simulink model "Final_Input_dat_rev1"  (R2024a)
settings: Solver=VariableStepAuto  StartTime=0.0  StopTime=10.0  RelTol=1e-3
libraries: CarMaker4SL x58
settings Model: Creator=namwoo.kim  LastModifiedBy=namwoo.kim

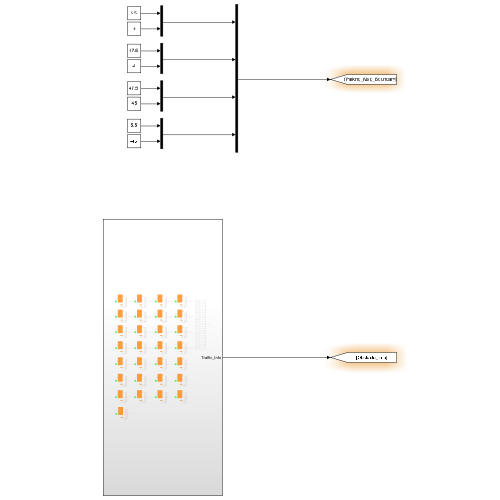
[thumbnail: Simulink's stored preview of the top-level diagram]
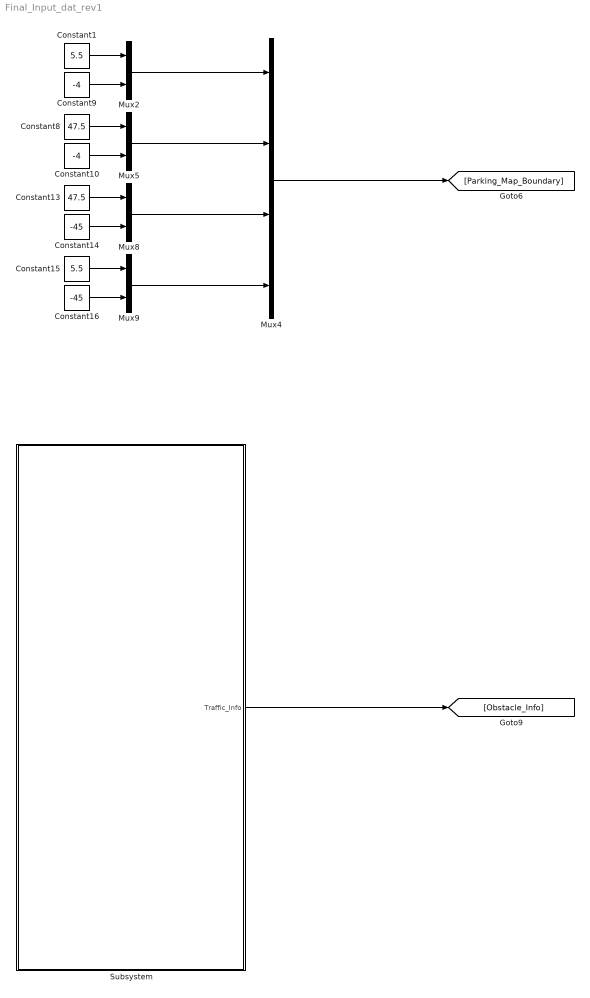
== system Final_Input_dat_rev1 ==
  Constant1 : Constant  Value=5.5
  Constant10 : Constant  Value=-4
  Constant13 : Constant  Value=47.5
  Constant14 : Constant  Value=-45
  Constant15 : Constant  Value=5.5
  Constant16 : Constant  Value=-45
  Constant8 : Constant  Value=47.5
  Constant9 : Constant  Value=-4
  Mux{2,5,8..9} (4 alike) : Mux  Inputs=2
  Mux4 : Mux
  Subsystem : Subsystem
  wires:
  Constant8/1 -> Mux5/1
  Constant16/1 -> Mux9/2
  Constant10/1 -> Mux5/2
  Mux4/1 -> [Parking_Map_Boundary]
  Constant15/1 -> Mux9/1
  Constant1/1 -> Mux2/1
  Mux8/1 -> Mux4/3
  Mux2/1 -> Mux4/1
  Mux5/1 -> Mux4/2
  Constant13/1 -> Mux8/1
  Constant9/1 -> Mux2/2
  Subsystem/1(Traffic_Info) -> [Obstacle_Info]
  Mux9/1 -> Mux4/4
  Constant14/1 -> Mux8/2

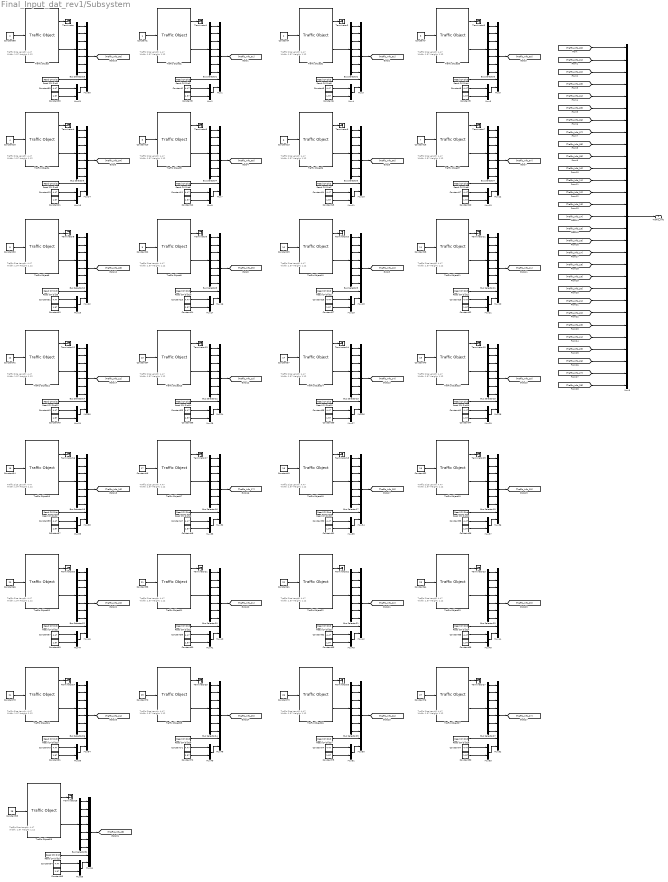
== system Final_Input_dat_rev1/Subsystem ==
  note: Traffic Size
      | Length: 4.47
      | Width: 1.97
      | Height: 1.12
  note: Traffic Size
      | Length: 4.47
      | Width: 1.97
      | Height: 1.12
  note: Traffic Size
      | Length: 4.47
      | Width: 1.97
      | Height: 1.12
  note: Traffic Size
      | Length: 4.47
      | Width: 1.97
      | Height: 1.12
  note: Traffic Size
      | Length: 4.47
      | Width: 1.97
      | Height: 1.12
  note: Traffic Size
      | Length: 4.47
      | Width: 1.97
      | Height: 1.12
  note: Traffic Size
      | Length: 4.47
      | Width: 1.97
      | Height: 1.12
  note: Traffic Size
      | Length: 4.47
      | Width: 1.97
      | Height: 1.12
  note: Traffic Size
      | Length: 4.47
      | Width: 1.97
      | Height: 1.12
  note: Traffic Size
      | Length: 4.47
      | Width: 1.97
      | Height: 1.12
  note: Traffic Size
      | Length: 4.47
      | Width: 1.97
      | Height: 1.12
  note: Traffic Size
      | Length: 4.47
      | Width: 1.97
      | Height: 1.12
  note: Traffic Size
      | Length: 4.47
      | Width: 1.97
      | Height: 1.12
  note: Traffic Size
      | Length: 4.47
      | Width: 1.97
      | Height: 1.12
  note: Traffic Size
      | Length: 4.47
      | Width: 1.97
      | Height: 1.12
  note: Traffic Size
      | Length: 4.47
      | Width: 1.97
      | Height: 1.12
  note: Traffic Size
      | Length: 4.47
      | Width: 1.97
      | Height: 1.12
  note: Traffic Size
      | Length: 4.47
      | Width: 1.97
      | Height: 1.12
  note: Traffic Size
      | Length: 4.47
      | Width: 1.97
      | Height: 1.12
  note: Traffic Size
      | Length: 4.47
      | Width: 1.97
      | Height: 1.12
  note: Traffic Size
      | Length: 4.47
      | Width: 1.97
      | Height: 1.12
  note: Traffic Size
      | Length: 4.47
      | Width: 1.97
      | Height: 1.12
  note: Traffic Size
      | Length: 4.47
      | Width: 1.97
      | Height: 1.12
  note: Traffic Size
      | Length: 4.47
      | Width: 1.97
      | Height: 1.12
  note: Traffic Size
      | Length: 4.47
      | Width: 1.97
      | Height: 1.12
  note: Traffic Size
      | Length: 4.47
      | Width: 1.97
      | Height: 1.12
  note: Traffic Size
      | Length: 4.47
      | Width: 1.97
      | Height: 1.12
  note: Traffic Size
      | Length: 4.47
      | Width: 1.97
      | Height: 1.12
  note: Traffic Size
      | Length: 4.47
      | Width: 1.97
      | Height: 1.12
  Bus Selector{1..27,29,31} (29 alike) : BusSelector  OutputSignals=t_0 x,t_0 y,v_0 x,v_0 y,a_0 x,a_0 y,r_zyx z
  Constant1 : Constant
  Constant10 : Constant  Value=5
  Constant{2,5,8,11,14,17,19,23,26,29,31,35,38,41,43,47,50,53,55,59,62,65,67,71,74,77,79,89,94} (29 alike) : Constant  Value=4.47
  Constant{3,6,9,12,15,20..21,24,27,32..33,36,39,44..45,48,51,56..57,60,63,68..69,72,75,80..81,90,96} (29 alike) : Constant  Value=1.97
  Constant13 : Constant  Value=6
  Constant16 : Constant  Value=7
  Constant18 : Constant  Value=4
  Constant22 : Constant  Value=9
  Constant25 : Constant  Value=10
  Constant28 : Constant  Value=11
  Constant30 : Constant  Value=8
  Constant34 : Constant  Value=13
  Constant37 : Constant  Value=14
  Constant4 : Constant  Value=2
  Constant40 : Constant  Value=15
  Constant42 : Constant  Value=12
  Constant46 : Constant  Value=17
  Constant49 : Constant  Value=18
  Constant52 : Constant  Value=19
  Constant54 : Constant  Value=16
  Constant58 : Constant  Value=21
  Constant61 : Constant  Value=22
  Constant64 : Constant  Value=23
  Constant66 : Constant  Value=20
  Constant7 : Constant  Value=3
  Constant70 : Constant  Value=25
  Constant73 : Constant  Value=26
  Constant76 : Constant  Value=27
  Constant78 : Constant  Value=24
  Constant88 : Constant  Value=0
  Constant93 : Constant  Value=28
  Mux{1,3,5,7,10,12,14,16,18,20,22,24,26,28,30,32,34,36,38,40,42,44,46,48,50,52,54,60,64} (29 alike) : Mux  Inputs=9
  Mux{2,4,6,8,11,13,15,17,19,21,23,25,27,29,31,33,35,37,39,41,43,45,47,49,51,53,55,61,65} (29 alike) : Mux  Inputs=2
  Mux9 : Mux  Inputs=29
  Read CM Dict1 : CarMaker4SL/Read CM Dict  xname=Traffic.T00.rzv  xsync=off  xstime=Inherited
  Read CM Dict10 : CarMaker4SL/Read CM Dict  xname=Traffic.T09.rzv  xsync=off  xstime=Inherited
  Read CM Dict11 : CarMaker4SL/Read CM Dict  xname=Traffic.T10.rzv  xsync=off  xstime=Inherited
  Read CM Dict12 : CarMaker4SL/Read CM Dict  xname=Traffic.T11.rzv  xsync=off  xstime=Inherited
  Read CM Dict13 : CarMaker4SL/Read CM Dict  xname=Traffic.T12.rzv  xsync=off  xstime=Inherited
  Read CM Dict14 : CarMaker4SL/Read CM Dict  xname=Traffic.T13.rzv  xsync=off  xstime=Inherited
  Read CM Dict15 : CarMaker4SL/Read CM Dict  xname=Traffic.T14.rzv  xsync=off  xstime=Inherited
  Read CM Dict16 : CarMaker4SL/Read CM Dict  xname=Traffic.T15.rzv  xsync=off  xstime=Inherited
  Read CM Dict17 : CarMaker4SL/Read CM Dict  xname=Traffic.T16.rzv  xsync=off  xstime=Inherited
  Read CM Dict18 : CarMaker4SL/Read CM Dict  xname=Traffic.T17.rzv  xsync=off  xstime=Inherited
  Read CM Dict19 : CarMaker4SL/Read CM Dict  xname=Traffic.T18.rzv  xsync=off  xstime=Inherited
  Read CM Dict2 : CarMaker4SL/Read CM Dict  xname=Traffic.T01.rzv  xsync=off  xstime=Inherited
  Read CM Dict20 : CarMaker4SL/Read CM Dict  xname=Traffic.T15.rzv  xsync=off  xstime=Inherited
  Read CM Dict21 : CarMaker4SL/Read CM Dict  xname=Traffic.T20.rzv  xsync=off  xstime=Inherited
  Read CM Dict22 : CarMaker4SL/Read CM Dict  xname=Traffic.T21.rzv  xsync=off  xstime=Inherited
  Read CM Dict23 : CarMaker4SL/Read CM Dict  xname=Traffic.T22.rzv  xsync=off  xstime=Inherited
  Read CM Dict24 : CarMaker4SL/Read CM Dict  xname=Traffic.T23.rzv  xsync=off  xstime=Inherited
  Read CM Dict25 : CarMaker4SL/Read CM Dict  xname=Traffic.T24.rzv  xsync=off  xstime=Inherited
  Read CM Dict26 : CarMaker4SL/Read CM Dict  xname=Traffic.T25.rzv  xsync=off  xstime=Inherited
  Read CM Dict27 : CarMaker4SL/Read CM Dict  xname=Traffic.T26.rzv  xsync=off  xstime=Inherited
  Read CM Dict28 : CarMaker4SL/Read CM Dict  xname=Traffic.T27.rzv  xsync=off  xstime=Inherited
  Read CM Dict29 : CarMaker4SL/Read CM Dict  xname=Traffic.T28.rzv  xsync=off  xstime=Inherited
  Read CM Dict3 : CarMaker4SL/Read CM Dict  xname=Traffic.T02.rzv  xsync=off  xstime=Inherited
  Read CM Dict4 : CarMaker4SL/Read CM Dict  xname=Traffic.T03.rzv  xsync=off  xstime=Inherited
  Read CM Dict5 : CarMaker4SL/Read CM Dict  xname=Traffic.T04.rzv  xsync=off  xstime=Inherited
  Read CM Dict6 : CarMaker4SL/Read CM Dict  xname=Traffic.T05.rzv  xsync=off  xstime=Inherited
  Read CM Dict7 : CarMaker4SL/Read CM Dict  xname=Traffic.T06.rzv  xsync=off  xstime=Inherited
  Read CM Dict8 : CarMaker4SL/Read CM Dict  xname=Traffic.T07.rzv  xsync=off  xstime=Inherited
  Read CM Dict9 : CarMaker4SL/Read CM Dict  xname=Traffic.T08.rzv  xsync=off  xstime=Inherited
  Terminator{,1..28} (29 alike) : Terminator
  Traffic Object : CarMaker4SL/Traffic Object  xname=T00  ximode=Traffic Id  xstime=Inherited
      settings: SourceProductName=CarMaker4SL
  Traffic Object1 : CarMaker4SL/Traffic Object  xname=T01  ximode=Traffic Id  xstime=Inherited
      settings: SourceProductName=CarMaker4SL
  Traffic Object10 : CarMaker4SL/Traffic Object  xname=T10  ximode=Traffic Id  xstime=Inherited
      settings: SourceProductName=CarMaker4SL
  Traffic Object11 : CarMaker4SL/Traffic Object  xname=T11  ximode=Traffic Id  xstime=Inherited
      settings: SourceProductName=CarMaker4SL
  Traffic Object12 : CarMaker4SL/Traffic Object  xname=T12  ximode=Traffic Id  xstime=Inherited
      settings: SourceProductName=CarMaker4SL
  Traffic Object13 : CarMaker4SL/Traffic Object  xname=T13  ximode=Traffic Id  xstime=Inherited
      settings: SourceProductName=CarMaker4SL
  Traffic Object14 : CarMaker4SL/Traffic Object  xname=T14  ximode=Traffic Id  xstime=Inherited
      settings: SourceProductName=CarMaker4SL
  Traffic Object15 : CarMaker4SL/Traffic Object  xname=T15  ximode=Traffic Id  xstime=Inherited
      settings: SourceProductName=CarMaker4SL
  Traffic Object16 : CarMaker4SL/Traffic Object  xname=T16  ximode=Traffic Id  xstime=Inherited
      settings: SourceProductName=CarMaker4SL
  Traffic Object17 : CarMaker4SL/Traffic Object  xname=T17  ximode=Traffic Id  xstime=Inherited
      settings: SourceProductName=CarMaker4SL
  Traffic Object18 : CarMaker4SL/Traffic Object  xname=T18  ximode=Traffic Id  xstime=Inherited
      settings: SourceProductName=CarMaker4SL
  Traffic Object19 : CarMaker4SL/Traffic Object  xname=T19  ximode=Traffic Id  xstime=Inherited
      settings: SourceProductName=CarMaker4SL
  Traffic Object2 : CarMaker4SL/Traffic Object  xname=T02  ximode=Traffic Id  xstime=Inherited
      settings: SourceProductName=CarMaker4SL
  Traffic Object20 : CarMaker4SL/Traffic Object  xname=T20  ximode=Traffic Id  xstime=Inherited
      settings: SourceProductName=CarMaker4SL
  Traffic Object21 : CarMaker4SL/Traffic Object  xname=T21  ximode=Traffic Id  xstime=Inherited
      settings: SourceProductName=CarMaker4SL
  Traffic Object22 : CarMaker4SL/Traffic Object  xname=T22  ximode=Traffic Id  xstime=Inherited
      settings: SourceProductName=CarMaker4SL
  Traffic Object23 : CarMaker4SL/Traffic Object  xname=T23  ximode=Traffic Id  xstime=Inherited
      settings: SourceProductName=CarMaker4SL
  Traffic Object24 : CarMaker4SL/Traffic Object  xname=T24  ximode=Traffic Id  xstime=Inherited
      settings: SourceProductName=CarMaker4SL
  Traffic Object25 : CarMaker4SL/Traffic Object  xname=T25  ximode=Traffic Id  xstime=Inherited
      settings: SourceProductName=CarMaker4SL
  Traffic Object26 : CarMaker4SL/Traffic Object  xname=T26  ximode=Traffic Id  xstime=Inherited
      settings: SourceProductName=CarMaker4SL
  Traffic Object27 : CarMaker4SL/Traffic Object  xname=T27  ximode=Traffic Id  xstime=Inherited
      settings: SourceProductName=CarMaker4SL
  Traffic Object28 : CarMaker4SL/Traffic Object  xname=T28  ximode=Traffic Id  xstime=Inherited
      settings: SourceProductName=CarMaker4SL
  Traffic Object3 : CarMaker4SL/Traffic Object  xname=T03  ximode=Traffic Id  xstime=Inherited
      settings: SourceProductName=CarMaker4SL
  Traffic Object4 : CarMaker4SL/Traffic Object  xname=T04  ximode=Traffic Id  xstime=Inherited
      settings: SourceProductName=CarMaker4SL
  Traffic Object5 : CarMaker4SL/Traffic Object  xname=T05  ximode=Traffic Id  xstime=Inherited
      settings: SourceProductName=CarMaker4SL
  Traffic Object6 : CarMaker4SL/Traffic Object  xname=T06  ximode=Traffic Id  xstime=Inherited
      settings: SourceProductName=CarMaker4SL
  Traffic Object7 : CarMaker4SL/Traffic Object  xname=T07  ximode=Traffic Id  xstime=Inherited
      settings: SourceProductName=CarMaker4SL
  Traffic Object8 : CarMaker4SL/Traffic Object  xname=T08  ximode=Traffic Id  xstime=Inherited
      settings: SourceProductName=CarMaker4SL
  Traffic Object9 : CarMaker4SL/Traffic Object  xname=T09  ximode=Traffic Id  xstime=Inherited
      settings: SourceProductName=CarMaker4SL
  Traffic_Info : Outport
  wires:
  [Traffic_Info_00] -> Mux9/1
  [Traffic_Info_01] -> Mux9/2
  Mux9/1 -> Traffic_Info/1
  [Traffic_Info_02] -> Mux9/3
  [Traffic_Info_06] -> Mux9/7
  [Traffic_Info_05] -> Mux9/6
  [Traffic_Info_04] -> Mux9/5
  [Traffic_Info_03] -> Mux9/4
  [Traffic_Info_09] -> Mux9/10
  [Traffic_Info_10] -> Mux9/11
  [Traffic_Info_11] -> Mux9/12
  [Traffic_Info_08] -> Mux9/9
  [Traffic_Info_12] -> Mux9/13
  [Traffic_Info_13] -> Mux9/14
  [Traffic_Info_07] -> Mux9/8
  [Traffic_Info_16] -> Mux9/17
  [Traffic_Info_17] -> Mux9/18
  [Traffic_Info_18] -> Mux9/19
  [Traffic_Info_15] -> Mux9/16
  [Traffic_Info_19] -> Mux9/20
  [Traffic_Info_20] -> Mux9/21
  [Traffic_Info_14] -> Mux9/15
  [Traffic_Info_23] -> Mux9/24
  [Traffic_Info_24] -> Mux9/25
  [Traffic_Info_25] -> Mux9/26
  [Traffic_Info_22] -> Mux9/23
  [Traffic_Info_26] -> Mux9/27
  [Traffic_Info_27] -> Mux9/28
  [Traffic_Info_21] -> Mux9/22
  [Traffic_Info_28] -> Mux9/29
  Traffic Object/2 -> Bus Selector29/1
  Constant88/1 -> Traffic Object/1
  Traffic Object/1 -> Terminator/1
  Bus Selector29/1 -> Mux60/1  "<t_0 x>"
  Bus Selector29/2 -> Mux60/2  "<t_0 y>"
  Bus Selector29/4 -> Mux60/4  "<v_0 y>"
  Bus Selector29/5 -> Mux60/5  "<a_0 x>"
  Bus Selector29/3 -> Mux60/3  "<v_0 x>"
  Bus Selector29/6 -> Mux60/6  "<a_0 y>"
  Bus Selector29/7 -> Mux60/7  "<r_zyx z>"
  Read CM Dict1/1 -> Mux60/8
  Mux60/1 -> [Traffic_Info_00]
  Constant89/1 -> Mux61/1
  Constant90/1 -> Mux61/2
  Mux61/1 -> Mux60/9
  Mux2/1 -> Mux1/9
  Constant2/1 -> Mux2/1
  Constant3/1 -> Mux2/2
  Bus Selector1/2 -> Mux1/2  "<t_0 y>"
  Traffic Object1/2 -> Bus Selector1/1
  Traffic Object1/1 -> Terminator1/1
  Constant1/1 -> Traffic Object1/1
  Read CM Dict2/1 -> Mux1/8
  Bus Selector1/1 -> Mux1/1  "<t_0 x>"
  Bus Selector1/6 -> Mux1/6  "<a_0 y>"
  Bus Selector1/7 -> Mux1/7  "<r_zyx z>"
  Bus Selector1/4 -> Mux1/4  "<v_0 y>"
  Bus Selector1/5 -> Mux1/5  "<a_0 x>"
  Mux1/1 -> [Traffic_Info_01]
  Bus Selector1/3 -> Mux1/3  "<v_0 x>"
  Mux4/1 -> Mux3/9
  Constant5/1 -> Mux4/1
  Constant6/1 -> Mux4/2
  Bus Selector2/2 -> Mux3/2  "<t_0 y>"
  Traffic Object2/2 -> Bus Selector2/1
  Traffic Object2/1 -> Terminator2/1
  Constant4/1 -> Traffic Object2/1
  Read CM Dict3/1 -> Mux3/8
  Bus Selector2/1 -> Mux3/1  "<t_0 x>"
  Bus Selector2/6 -> Mux3/6  "<a_0 y>"
  Bus Selector2/7 -> Mux3/7  "<r_zyx z>"
  Bus Selector2/4 -> Mux3/4  "<v_0 y>"
  Bus Selector2/5 -> Mux3/5  "<a_0 x>"
  Mux3/1 -> [Traffic_Info_02]
  Bus Selector2/3 -> Mux3/3  "<v_0 x>"
  Mux6/1 -> Mux5/9
  Constant8/1 -> Mux6/1
  Constant9/1 -> Mux6/2
  Bus Selector3/2 -> Mux5/2  "<t_0 y>"
  Traffic Object3/2 -> Bus Selector3/1
  Traffic Object3/1 -> Terminator3/1
  Constant7/1 -> Traffic Object3/1
  Read CM Dict4/1 -> Mux5/8
  Bus Selector3/1 -> Mux5/1  "<t_0 x>"
  Bus Selector3/6 -> Mux5/6  "<a_0 y>"
  Bus Selector3/7 -> Mux5/7  "<r_zyx z>"
  Bus Selector3/4 -> Mux5/4  "<v_0 y>"
  Bus Selector3/5 -> Mux5/5  "<a_0 x>"
  Mux5/1 -> [Traffic_Info_03]
  Bus Selector3/3 -> Mux5/3  "<v_0 x>"
  Constant19/1 -> Mux15/1
  Constant21/1 -> Mux15/2
  Bus Selector4/3 -> Mux7/3  "<v_0 x>"
  Bus Selector4/4 -> Mux7/4  "<v_0 y>"
  Bus Selector4/7 -> Mux7/7  "<r_zyx z>"
  Read CM Dict6/1 -> Mux7/8
  Traffic Object5/1 -> Terminator5/1
  Mux15/1 -> Mux14/9
  Bus Selector4/2 -> Mux7/2  "<t_0 y>"
  Constant11/1 -> Mux8/1
  Constant12/1 -> Mux8/2
  Bus Selector4/1 -> Mux7/1  "<t_0 x>"
  Bus Selector5/3 -> Mux10/3  "<v_0 x>"
  Bus Selector5/4 -> Mux10/4  "<v_0 y>"
  Bus Selector5/7 -> Mux10/7  "<r_zyx z>"
  Traffic Object4/1 -> Terminator4/1
  Constant18/1 -> Traffic Object4/1
  Bus Selector5/1 -> Mux10/1  "<t_0 x>"
  Bus Selector5/6 -> Mux10/6  "<a_0 y>"
  Traffic Object4/2 -> Bus Selector6/1
  Bus Selector7/3 -> Mux12/3  "<v_0 x>"
  Bus Selector6/2 -> Mux14/2  "<t_0 y>"
  Mux7/1 -> [Traffic_Info_05]
  Bus Selector7/4 -> Mux12/4  "<v_0 y>"
  Mux12/1 -> [Traffic_Info_07]
  Traffic Object7/2 -> Bus Selector7/1
  Read CM Dict8/1 -> Mux12/8
  Constant16/1 -> Traffic Object7/1
  Read CM Dict5/1 -> Mux14/8
  Mux13/1 -> Mux12/9
  Bus Selector4/6 -> Mux7/6  "<a_0 y>"
  Constant20/1 -> Mux13/2
  Constant10/1 -> Traffic Object5/1
  Bus Selector7/7 -> Mux12/7  "<r_zyx z>"
  Traffic Object5/2 -> Bus Selector4/1
  Traffic Object7/1 -> Terminator7/1
  Bus Selector6/1 -> Mux14/1  "<t_0 x>"
  Bus Selector6/7 -> Mux14/7  "<r_zyx z>"
  Bus Selector7/6 -> Mux12/6  "<a_0 y>"
  Bus Selector6/4 -> Mux14/4  "<v_0 y>"
  Constant13/1 -> Traffic Object6/1
  Bus Selector5/5 -> Mux10/5  "<a_0 x>"
  Traffic Object6/1 -> Terminator6/1
  Read CM Dict7/1 -> Mux10/8
  Bus Selector5/2 -> Mux10/2  "<t_0 y>"
  Bus Selector7/1 -> Mux12/1  "<t_0 x>"
  Constant14/1 -> Mux11/1
  Bus Selector7/2 -> Mux12/2  "<t_0 y>"
  Mux8/1 -> Mux7/9
  Constant15/1 -> Mux11/2
  Bus Selector4/5 -> Mux7/5  "<a_0 x>"
  Traffic Object6/2 -> Bus Selector5/1
  Bus Selector6/6 -> Mux14/6  "<a_0 y>"
  Bus Selector6/5 -> Mux14/5  "<a_0 x>"
  Bus Selector7/5 -> Mux12/5  "<a_0 x>"
  Mux11/1 -> Mux10/9
  Mux14/1 -> [Traffic_Info_04]
  Constant17/1 -> Mux13/1
  Bus Selector6/3 -> Mux14/3  "<v_0 x>"
  Mux10/1 -> [Traffic_Info_06]
  Constant31/1 -> Mux23/1
  Constant33/1 -> Mux23/2
  Bus Selector8/3 -> Mux16/3  "<v_0 x>"
  Bus Selector8/4 -> Mux16/4  "<v_0 y>"
  Bus Selector8/7 -> Mux16/7  "<r_zyx z>"
  Read CM Dict10/1 -> Mux16/8
  Traffic Object9/1 -> Terminator9/1
  Mux23/1 -> Mux22/9
  Bus Selector8/2 -> Mux16/2  "<t_0 y>"
  Constant23/1 -> Mux17/1
  Constant24/1 -> Mux17/2
  Bus Selector8/1 -> Mux16/1  "<t_0 x>"
  Bus Selector9/3 -> Mux18/3  "<v_0 x>"
  Bus Selector9/4 -> Mux18/4  "<v_0 y>"
  Bus Selector9/7 -> Mux18/7  "<r_zyx z>"
  Traffic Object8/1 -> Terminator8/1
  Constant30/1 -> Traffic Object8/1
  Bus Selector9/1 -> Mux18/1  "<t_0 x>"
  Bus Selector9/6 -> Mux18/6  "<a_0 y>"
  Traffic Object8/2 -> Bus Selector10/1
  Bus Selector11/3 -> Mux20/3  "<v_0 x>"
  Bus Selector10/2 -> Mux22/2  "<t_0 y>"
  Mux16/1 -> [Traffic_Info_09]
  Bus Selector11/4 -> Mux20/4  "<v_0 y>"
  Mux20/1 -> [Traffic_Info_11]
  Traffic Object11/2 -> Bus Selector11/1
  Read CM Dict12/1 -> Mux20/8
  Constant28/1 -> Traffic Object11/1
  Read CM Dict9/1 -> Mux22/8
  Mux21/1 -> Mux20/9
  Bus Selector8/6 -> Mux16/6  "<a_0 y>"
  Constant32/1 -> Mux21/2
  Constant22/1 -> Traffic Object9/1
  Bus Selector11/7 -> Mux20/7  "<r_zyx z>"
  Traffic Object9/2 -> Bus Selector8/1
  Traffic Object11/1 -> Terminator11/1
  Bus Selector10/1 -> Mux22/1  "<t_0 x>"
  Bus Selector10/7 -> Mux22/7  "<r_zyx z>"
  Bus Selector11/6 -> Mux20/6  "<a_0 y>"
  Bus Selector10/4 -> Mux22/4  "<v_0 y>"
  Constant25/1 -> Traffic Object10/1
  Bus Selector9/5 -> Mux18/5  "<a_0 x>"
  Traffic Object10/1 -> Terminator10/1
  Read CM Dict11/1 -> Mux18/8
  Bus Selector9/2 -> Mux18/2  "<t_0 y>"
  Bus Selector11/1 -> Mux20/1  "<t_0 x>"
  Constant26/1 -> Mux19/1
  Bus Selector11/2 -> Mux20/2  "<t_0 y>"
  Mux17/1 -> Mux16/9
  Constant27/1 -> Mux19/2
  Bus Selector8/5 -> Mux16/5  "<a_0 x>"
  Traffic Object10/2 -> Bus Selector9/1
  Bus Selector10/6 -> Mux22/6  "<a_0 y>"
  Bus Selector10/5 -> Mux22/5  "<a_0 x>"
  Bus Selector11/5 -> Mux20/5  "<a_0 x>"
  Mux19/1 -> Mux18/9
  Mux22/1 -> [Traffic_Info_08]
  Constant29/1 -> Mux21/1
  Bus Selector10/3 -> Mux22/3  "<v_0 x>"
  Mux18/1 -> [Traffic_Info_10]
  Constant43/1 -> Mux31/1
  Constant45/1 -> Mux31/2
  Bus Selector12/3 -> Mux24/3  "<v_0 x>"
  Bus Selector12/4 -> Mux24/4  "<v_0 y>"
  Bus Selector12/7 -> Mux24/7  "<r_zyx z>"
  Read CM Dict14/1 -> Mux24/8
  Traffic Object13/1 -> Terminator13/1
  Mux31/1 -> Mux30/9
  Bus Selector12/2 -> Mux24/2  "<t_0 y>"
  Constant35/1 -> Mux25/1
  Constant36/1 -> Mux25/2
  Bus Selector12/1 -> Mux24/1  "<t_0 x>"
  Bus Selector13/3 -> Mux26/3  "<v_0 x>"
  Bus Selector13/4 -> Mux26/4  "<v_0 y>"
  Bus Selector13/7 -> Mux26/7  "<r_zyx z>"
  Traffic Object12/1 -> Terminator12/1
  Constant42/1 -> Traffic Object12/1
  Bus Selector13/1 -> Mux26/1  "<t_0 x>"
  Bus Selector13/6 -> Mux26/6  "<a_0 y>"
  Traffic Object12/2 -> Bus Selector14/1
  Bus Selector15/3 -> Mux28/3  "<v_0 x>"
  Bus Selector14/2 -> Mux30/2  "<t_0 y>"
  Mux24/1 -> [Traffic_Info_13]
  Bus Selector15/4 -> Mux28/4  "<v_0 y>"
  Mux28/1 -> [Traffic_Info_15]
  Traffic Object15/2 -> Bus Selector15/1
  Read CM Dict16/1 -> Mux28/8
  Constant40/1 -> Traffic Object15/1
  Read CM Dict13/1 -> Mux30/8
  Mux29/1 -> Mux28/9
  Bus Selector12/6 -> Mux24/6  "<a_0 y>"
  Constant44/1 -> Mux29/2
  Constant34/1 -> Traffic Object13/1
  Bus Selector15/7 -> Mux28/7  "<r_zyx z>"
  Traffic Object13/2 -> Bus Selector12/1
  Traffic Object15/1 -> Terminator15/1
  Bus Selector14/1 -> Mux30/1  "<t_0 x>"
  Bus Selector14/7 -> Mux30/7  "<r_zyx z>"
  Bus Selector15/6 -> Mux28/6  "<a_0 y>"
  Bus Selector14/4 -> Mux30/4  "<v_0 y>"
  Constant37/1 -> Traffic Object14/1
  Bus Selector13/5 -> Mux26/5  "<a_0 x>"
  Traffic Object14/1 -> Terminator14/1
  Read CM Dict15/1 -> Mux26/8
  Bus Selector13/2 -> Mux26/2  "<t_0 y>"
  Bus Selector15/1 -> Mux28/1  "<t_0 x>"
  Constant38/1 -> Mux27/1
  Bus Selector15/2 -> Mux28/2  "<t_0 y>"
  Mux25/1 -> Mux24/9
  Constant39/1 -> Mux27/2
  Bus Selector12/5 -> Mux24/5  "<a_0 x>"
  Traffic Object14/2 -> Bus Selector13/1
  Bus Selector14/6 -> Mux30/6  "<a_0 y>"
  Bus Selector14/5 -> Mux30/5  "<a_0 x>"
  Bus Selector15/5 -> Mux28/5  "<a_0 x>"
  Mux27/1 -> Mux26/9
  Mux30/1 -> [Traffic_Info_12]
  Constant41/1 -> Mux29/1
  Bus Selector14/3 -> Mux30/3  "<v_0 x>"
  Mux26/1 -> [Traffic_Info_14]
  Bus Selector18/3 -> Mux38/3  "<v_0 x>"
  Bus Selector19/5 -> Mux36/5  "<a_0 x>"
  Bus Selector18/5 -> Mux38/5  "<a_0 x>"
  Traffic Object18/2 -> Bus Selector17/1
  Bus Selector18/6 -> Mux38/6  "<a_0 y>"
  Mux33/1 -> Mux32/9
  Constant51/1 -> Mux35/2
  Bus Selector19/2 -> Mux36/2  "<t_0 y>"
  Bus Selector17/2 -> Mux34/2  "<t_0 y>"
  Bus Selector17/5 -> Mux34/5  "<a_0 x>"
  Traffic Object18/1 -> Terminator18/1
  Bus Selector19/6 -> Mux36/6  "<a_0 y>"
  Bus Selector18/7 -> Mux38/7  "<r_zyx z>"
  Bus Selector19/7 -> Mux36/7  "<r_zyx z>"
  Bus Selector18/1 -> Mux38/1  "<t_0 x>"
  Traffic Object19/1 -> Terminator19/1
  Traffic Object19/2 -> Bus Selector19/1
  Constant56/1 -> Mux37/2
  Mux37/1 -> Mux36/9
  Constant49/1 -> Traffic Object18/1
  Read CM Dict20/1 -> Mux36/8
  Mux34/1 -> [Traffic_Info_18]
  Mux32/1 -> [Traffic_Info_17]
  Mux36/1 -> [Traffic_Info_19]
  Bus Selector19/4 -> Mux36/4  "<v_0 y>"
  Constant54/1 -> Traffic Object16/1
  Traffic Object16/1 -> Terminator16/1
  Bus Selector17/6 -> Mux34/6  "<a_0 y>"
  Bus Selector16/6 -> Mux32/6  "<a_0 y>"
  Bus Selector17/3 -> Mux34/3  "<v_0 x>"
  Read CM Dict17/1 -> Mux38/8
  Bus Selector17/4 -> Mux34/4  "<v_0 y>"
  Bus Selector18/4 -> Mux38/4  "<v_0 y>"
  Bus Selector17/1 -> Mux34/1  "<t_0 x>"
  Constant46/1 -> Traffic Object17/1
  Bus Selector17/7 -> Mux34/7  "<r_zyx z>"
  Constant53/1 -> Mux37/1
  Bus Selector18/2 -> Mux38/2  "<t_0 y>"
  Bus Selector16/1 -> Mux32/1  "<t_0 x>"
  Bus Selector19/1 -> Mux36/1  "<t_0 x>"
  Bus Selector16/3 -> Mux32/3  "<v_0 x>"
  Mux38/1 -> [Traffic_Info_16]
  Constant48/1 -> Mux33/2
  Traffic Object17/2 -> Bus Selector16/1
  Read CM Dict18/1 -> Mux32/8
  Bus Selector16/5 -> Mux32/5  "<a_0 x>"
  Traffic Object17/1 -> Terminator17/1
  Constant57/1 -> Mux39/2
  Bus Selector16/2 -> Mux32/2  "<t_0 y>"
  Bus Selector19/3 -> Mux36/3  "<v_0 x>"
  Constant52/1 -> Traffic Object19/1
  Bus Selector16/7 -> Mux32/7  "<r_zyx z>"
  Traffic Object16/2 -> Bus Selector18/1
  Read CM Dict19/1 -> Mux34/8
  Mux39/1 -> Mux38/9
  Constant50/1 -> Mux35/1
  Bus Selector16/4 -> Mux32/4  "<v_0 y>"
  Constant47/1 -> Mux33/1
  Constant55/1 -> Mux39/1
  Mux35/1 -> Mux34/9
  Bus Selector22/3 -> Mux46/3  "<v_0 x>"
  Bus Selector23/5 -> Mux44/5  "<a_0 x>"
  Bus Selector22/5 -> Mux46/5  "<a_0 x>"
  Traffic Object22/2 -> Bus Selector21/1
  Bus Selector22/6 -> Mux46/6  "<a_0 y>"
  Mux41/1 -> Mux40/9
  Constant63/1 -> Mux43/2
  Bus Selector23/2 -> Mux44/2  "<t_0 y>"
  Bus Selector21/2 -> Mux42/2  "<t_0 y>"
  Bus Selector21/5 -> Mux42/5  "<a_0 x>"
  Traffic Object22/1 -> Terminator22/1
  Bus Selector23/6 -> Mux44/6  "<a_0 y>"
  Bus Selector22/7 -> Mux46/7  "<r_zyx z>"
  Bus Selector23/7 -> Mux44/7  "<r_zyx z>"
  Bus Selector22/1 -> Mux46/1  "<t_0 x>"
  Traffic Object23/1 -> Terminator23/1
  Traffic Object23/2 -> Bus Selector23/1
  Constant68/1 -> Mux45/2
  Mux45/1 -> Mux44/9
  Constant61/1 -> Traffic Object22/1
  Read CM Dict24/1 -> Mux44/8
  Mux42/1 -> [Traffic_Info_22]
  Mux40/1 -> [Traffic_Info_21]
  Mux44/1 -> [Traffic_Info_23]
  Bus Selector23/4 -> Mux44/4  "<v_0 y>"
  Constant66/1 -> Traffic Object20/1
  Traffic Object20/1 -> Terminator20/1
  Bus Selector21/6 -> Mux42/6  "<a_0 y>"
  Bus Selector20/6 -> Mux40/6  "<a_0 y>"
  Bus Selector21/3 -> Mux42/3  "<v_0 x>"
  Read CM Dict21/1 -> Mux46/8
  Bus Selector21/4 -> Mux42/4  "<v_0 y>"
  Bus Selector22/4 -> Mux46/4  "<v_0 y>"
  Bus Selector21/1 -> Mux42/1  "<t_0 x>"
  Constant58/1 -> Traffic Object21/1
  Bus Selector21/7 -> Mux42/7  "<r_zyx z>"
  Constant65/1 -> Mux45/1
  Bus Selector22/2 -> Mux46/2  "<t_0 y>"
  Bus Selector20/1 -> Mux40/1  "<t_0 x>"
  Bus Selector23/1 -> Mux44/1  "<t_0 x>"
  Bus Selector20/3 -> Mux40/3  "<v_0 x>"
  Mux46/1 -> [Traffic_Info_20]
  Constant60/1 -> Mux41/2
  Traffic Object21/2 -> Bus Selector20/1
  Read CM Dict22/1 -> Mux40/8
  Bus Selector20/5 -> Mux40/5  "<a_0 x>"
  Traffic Object21/1 -> Terminator21/1
  Constant69/1 -> Mux47/2
  Bus Selector20/2 -> Mux40/2  "<t_0 y>"
  Bus Selector23/3 -> Mux44/3  "<v_0 x>"
  Constant64/1 -> Traffic Object23/1
  Bus Selector20/7 -> Mux40/7  "<r_zyx z>"
  Traffic Object20/2 -> Bus Selector22/1
  Read CM Dict23/1 -> Mux42/8
  Mux47/1 -> Mux46/9
  Constant62/1 -> Mux43/1
  Bus Selector20/4 -> Mux40/4  "<v_0 y>"
  Constant59/1 -> Mux41/1
  Constant67/1 -> Mux47/1
  Mux43/1 -> Mux42/9
  Bus Selector26/3 -> Mux54/3  "<v_0 x>"
  Bus Selector27/5 -> Mux52/5  "<a_0 x>"
  Bus Selector26/5 -> Mux54/5  "<a_0 x>"
  Traffic Object26/2 -> Bus Selector25/1
  Bus Selector26/6 -> Mux54/6  "<a_0 y>"
  Mux49/1 -> Mux48/9
  Constant75/1 -> Mux51/2
  Bus Selector27/2 -> Mux52/2  "<t_0 y>"
  Bus Selector25/2 -> Mux50/2  "<t_0 y>"
  Bus Selector25/5 -> Mux50/5  "<a_0 x>"
  Traffic Object26/1 -> Terminator26/1
  Bus Selector27/6 -> Mux52/6  "<a_0 y>"
  Bus Selector26/7 -> Mux54/7  "<r_zyx z>"
  Bus Selector27/7 -> Mux52/7  "<r_zyx z>"
  Bus Selector26/1 -> Mux54/1  "<t_0 x>"
  Traffic Object27/1 -> Terminator27/1
  Traffic Object27/2 -> Bus Selector27/1
  Constant80/1 -> Mux53/2
  Mux53/1 -> Mux52/9
  Constant73/1 -> Traffic Object26/1
  Read CM Dict28/1 -> Mux52/8
  Mux50/1 -> [Traffic_Info_26]
  Mux48/1 -> [Traffic_Info_25]
  Mux52/1 -> [Traffic_Info_27]
  Bus Selector27/4 -> Mux52/4  "<v_0 y>"
  Constant78/1 -> Traffic Object24/1
  Traffic Object24/1 -> Terminator24/1
  Bus Selector25/6 -> Mux50/6  "<a_0 y>"
  Bus Selector24/6 -> Mux48/6  "<a_0 y>"
  Bus Selector25/3 -> Mux50/3  "<v_0 x>"
  Read CM Dict25/1 -> Mux54/8
  Bus Selector25/4 -> Mux50/4  "<v_0 y>"
  Bus Selector26/4 -> Mux54/4  "<v_0 y>"
  Bus Selector25/1 -> Mux50/1  "<t_0 x>"
  Constant70/1 -> Traffic Object25/1
  Bus Selector25/7 -> Mux50/7  "<r_zyx z>"
  Constant77/1 -> Mux53/1
  Bus Selector26/2 -> Mux54/2  "<t_0 y>"
  Bus Selector24/1 -> Mux48/1  "<t_0 x>"
  Bus Selector27/1 -> Mux52/1  "<t_0 x>"
  Bus Selector24/3 -> Mux48/3  "<v_0 x>"
  Mux54/1 -> [Traffic_Info_24]
  Constant72/1 -> Mux49/2
  Traffic Object25/2 -> Bus Selector24/1
  Read CM Dict26/1 -> Mux48/8
  Bus Selector24/5 -> Mux48/5  "<a_0 x>"
  Traffic Object25/1 -> Terminator25/1
  Constant81/1 -> Mux55/2
  Bus Selector24/2 -> Mux48/2  "<t_0 y>"
  Bus Selector27/3 -> Mux52/3  "<v_0 x>"
  Constant76/1 -> Traffic Object27/1
  Bus Selector24/7 -> Mux48/7  "<r_zyx z>"
  Traffic Object24/2 -> Bus Selector26/1
  Read CM Dict27/1 -> Mux50/8
  Mux55/1 -> Mux54/9
  Constant74/1 -> Mux51/1
  Bus Selector24/4 -> Mux48/4  "<v_0 y>"
  Constant71/1 -> Mux49/1
  Constant79/1 -> Mux55/1
  Mux51/1 -> Mux50/9
  Bus Selector31/3 -> Mux64/3  "<v_0 x>"
  Bus Selector31/5 -> Mux64/5  "<a_0 x>"
  Bus Selector31/6 -> Mux64/6  "<a_0 y>"
  Bus Selector31/7 -> Mux64/7  "<r_zyx z>"
  Bus Selector31/1 -> Mux64/1  "<t_0 x>"
  Constant93/1 -> Traffic Object28/1
  Traffic Object28/1 -> Terminator28/1
  Read CM Dict29/1 -> Mux64/8
  Bus Selector31/4 -> Mux64/4  "<v_0 y>"
  Bus Selector31/2 -> Mux64/2  "<t_0 y>"
  Mux64/1 -> [Traffic_Info_28]
  Constant96/1 -> Mux65/2
  Traffic Object28/2 -> Bus Selector31/1
  Mux65/1 -> Mux64/9
  Constant94/1 -> Mux65/1
